simulink model "family_4_variant_2_MeasureMag"  (R2015a)
settings: configuration reference "AR_Drone_ConfigSet" (kept outside this file)
libraries: simulink x1, AR_Drone_2_Library x1
settings Model: SimulationMode=external  CovSFcnEnable=off  ExtModeTrigDuration=480000  Creator=darenlee  LastModifiedBy=Raphaël
settings ConfigSetRef: SourceLocation=Base Workspace

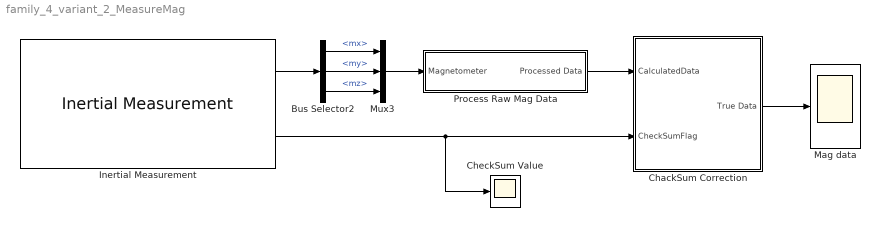
== system family_4_variant_2_MeasureMag ==
  Bus Selector2 : BusSelector  OutputSignals=mx,my,mz
  ChackSum Correction : Subsystem
  CheckSum Value : Scope
      settings: YMin=0  YMax=2500  SaveName=CheckSum1
  Inertial Measurement : AR_Drone_2_Library/Inertial Measurement  Ts=1/400
  Mag data : Scope
      settings: ShowLegends=on  TimeRange=100  YMin=-125  YMax=150  SaveName=MagData
  Mux3 : Mux  Inputs=3
  Process Raw Mag Data : Subsystem
  wires:
  Bus Selector2/1 -> Mux3/1  "<mx>"
  Bus Selector2/2 -> Mux3/2  "<my>"
  Bus Selector2/3 -> Mux3/3  "<mz>"
  Mux3/1 -> Process Raw Mag Data/1(Magnetometer)
  Inertial Measurement/2 -> ChackSum Correction/2(CheckSumFlag), CheckSum Value/1
  Process Raw Mag Data/1(Processed Data) -> ChackSum Correction/1(CalculatedData)
  Inertial Measurement/1 -> Bus Selector2/1
  ChackSum Correction/1(True Data) -> Mag data/1

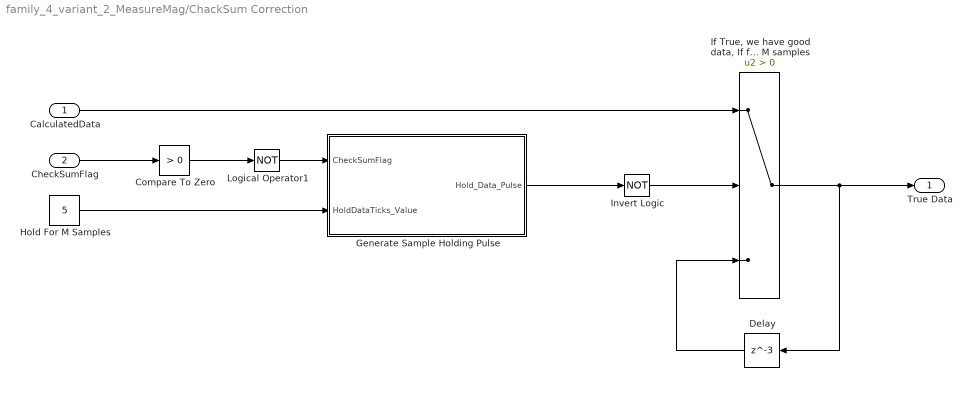
== system family_4_variant_2_MeasureMag/ChackSum Correction ==
  CalculatedData : Inport
  CheckSumFlag : Inport  Port=2
  Compare To Zero : simulink/Logic and Bit Operations/Compare To Zero  relop=>  OutDataTypeStr=boolean
  Delay : Delay  DelayLength=3  InitialCondition=0
  Generate Sample Holding Pulse : Subsystem
  Hold For M Samples : Constant  Value=5
  "If True, we have good data, If false, we have bad data, With bad data, use previous good data from N samples ago and hold it on that value for M samples" : Switch  Criteria=u2 > Threshold
  Invert Logic : Logic  Operator=NOT  AllPortsSameDT=off  OutDataTypeStr=boolean
  Logical Operator1 : Logic  Operator=NOT  AllPortsSameDT=off  OutDataTypeStr=boolean
  True Data : Outport
  wires:
  "If True, we have good data, If false, we have bad data, With bad data, use previous good data from N samples ago and hold it on that value for M samples"/1 -> Delay/1, True Data/1
  Delay/1 -> "If True, we have good data, If false, we have bad data, With bad data, use previous good data from N samples ago and hold it on that value for M samples"/3
  Invert Logic/1 -> "If True, we have good data, If false, we have bad data, With bad data, use previous good data from N samples ago and hold it on that value for M samples"/2
  Generate Sample Holding Pulse/1(Hold_Data_Pulse) -> Invert Logic/1
  Logical Operator1/1 -> Generate Sample Holding Pulse/1(CheckSumFlag)
  Compare To Zero/1 -> Logical Operator1/1
  Hold For M Samples/1 -> Generate Sample Holding Pulse/2(HoldDataTicks_Value)
  CheckSumFlag/1 -> Compare To Zero/1
  CalculatedData/1 -> "If True, we have good data, If false, we have bad data, With bad data, use previous good data from N samples ago and hold it on that value for M samples"/1

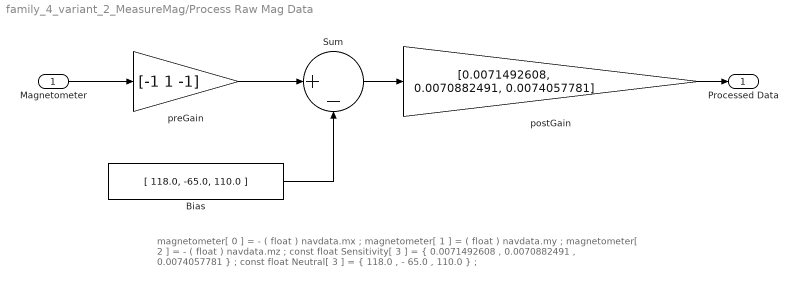
== system family_4_variant_2_MeasureMag/Process Raw Mag Data ==
  note: magnetometer[ 0 ] = - ( float ) navdata.mx ;
      | magnetometer[ 1 ] = ( float ) navdata.my ;
      | magnetometer[ 2 ] = - ( float ) navdata.mz ;
      | const float Sensitivity[ 3 ] = { 0.0071492608 , 0.0070882491 , 0.0074057781 } ;
      | const float Neutral[ 3 ] = { 118.0 , - 65.0 , 110.0 } ;
  Magnetometer : Inport
  Bias : Constant  Value=[ 118.0, -65.0, 110.0 ]
  Sum : Sum  Inputs=|+-
  postGain : Gain  Gain=[0.0071492608, 0.0070882491, 0.0074057781]
  preGain : Gain  Gain=[-1 1 -1]
  Processed Data : Outport
  wires:
  postGain/1 -> Processed Data/1
  Magnetometer/1 -> preGain/1
  Sum/1 -> postGain/1
  preGain/1 -> Sum/1
  Bias/1 -> Sum/2

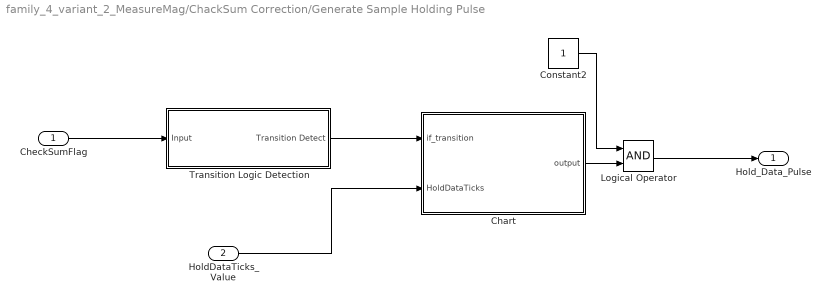
== system family_4_variant_2_MeasureMag/ChackSum Correction/Generate Sample Holding Pulse ==
  CheckSumFlag : Inport
  HoldDataTicks_Value : Inport  Port=2
  Chart : Stateflow chart  TreatAsAtomicUnit=on
  Constant2 : Constant
  Logical Operator : Logic  AllPortsSameDT=off  OutDataTypeStr=boolean
  Transition Logic Detection : Subsystem
  Hold_Data_Pulse : Outport
  wires:
  Constant2/1 -> Logical Operator/1
  Chart/1(output) -> Logical Operator/2
  Transition Logic Detection/1(Transition Detect) -> Chart/1(if_transition)
  CheckSumFlag/1 -> Transition Logic Detection/1(Input)
  HoldDataTicks_Value/1 -> Chart/2(HoldDataTicks)
  Logical Operator/1 -> Hold_Data_Pulse/1

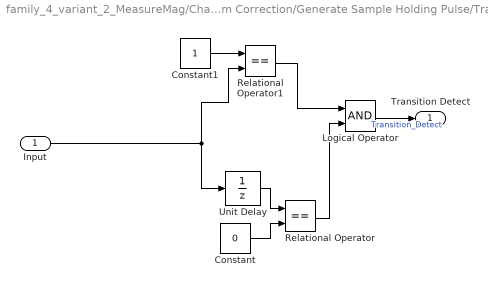
== system family_4_variant_2_MeasureMag/ChackSum Correction/Generate Sample Holding Pulse/Transition Logic Detection ==
  Input : Inport
  Constant : Constant  Value=0
  Constant1 : Constant
  Logical Operator : Logic  AllPortsSameDT=off  OutDataTypeStr=boolean
  Relational Operator : RelationalOperator  Operator===  OutDataTypeStr=boolean
  Relational Operator1 : RelationalOperator  Operator===  OutDataTypeStr=boolean
  Unit Delay : UnitDelay  SampleTime=-1
  Transition Detect : Outport
  wires:
  Relational Operator1/1 -> Logical Operator/1
  Unit Delay/1 -> Relational Operator/1
  Input/1 -> Relational Operator1/2, Unit Delay/1
  Relational Operator/1 -> Logical Operator/2
  Constant/1 -> Relational Operator/2
  Constant1/1 -> Relational Operator1/1
  Logical Operator/1 -> Transition Detect/1  "Transition_Detect"

== stateflow chart family_4_variant_2_MeasureMag/ChackSum Correction/Generate Sample Holding Pulse/Chart ==
  state Begin_State0
    entry: output =0;
  state Begin_State
    entry: output =1;
  state End_State
    entry: output=0;
  (default) -> Begin_State0
  Begin_State0 -> Begin_State : [if_transition==1]
  Begin_State -> End_State [order 1] : after(HoldDataTicks,tick)
  End_State -> Begin_State : [if_transition==1]
  Begin_State -> Begin_State [order 2] : [if_transition==1]
  data: output output; if_transition input; HoldDataTicks input
